simulink model "Transient_configuration_example_50_simscape"  (R2026a)
settings: Solver=ode23t  StopTime=120/60  EnableMultiTasking=on
undefined symbols (not defined in the file): Three_PhaseBreaker_class, Three_PhaseFault_class, Three_PhaseSeriesRLCLoad_class, Three_PhaseSource_class, Three_PhaseTransformer_1_class, Three_PhaseV_IMeasuremen_class
libraries: ee_lib x23, fl_lib x8, nesl_utility x8, eeRmsMeasurement x2
settings Model: Creator=Rodney Tan  LastModifiedBy=usuario
settings DebuggingCC: SaveWithParameterizedLinksMsg=none
settings SimscapeCC: SimscapeNormalizeSystem=off  SimscapeLogType=none  SimscapeLogDataHistory=5000.0

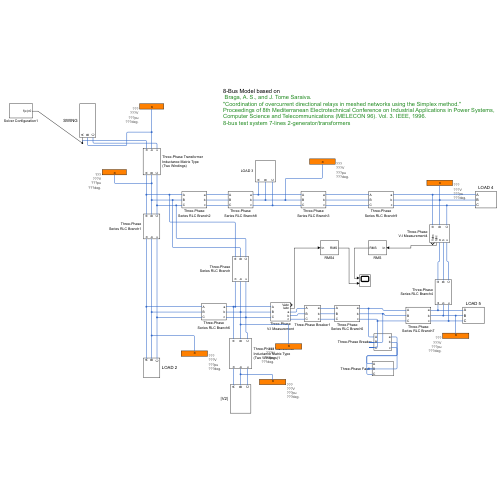
[thumbnail: Simulink's stored preview of the top-level diagram]
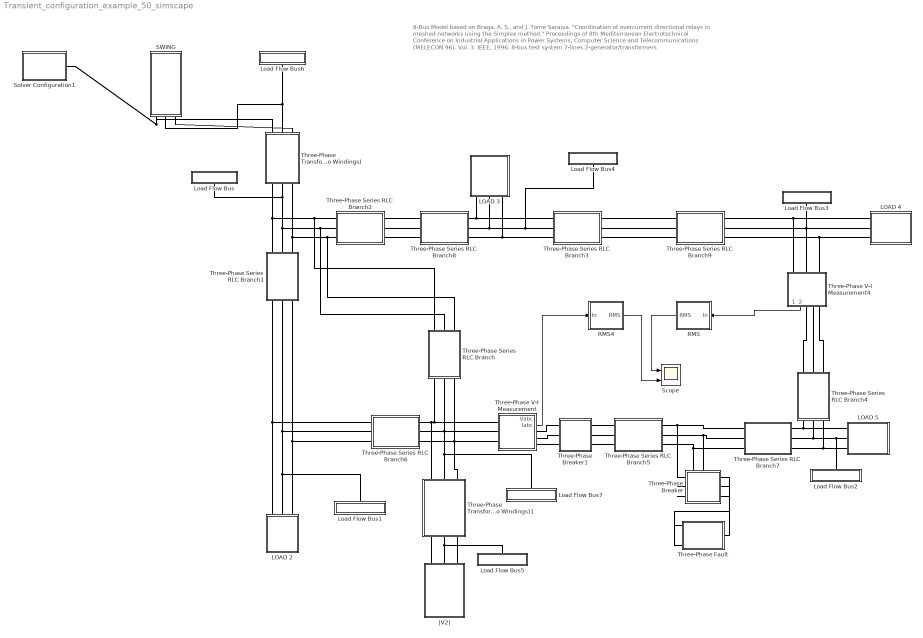
== system Transient_configuration_example_50_simscape ==
  note: 8-Bus Model based on
      | Braga, A. S., and J. Tome Saraiva.
      | "Coordination of overcurrent directional relays in meshed networks using the Simplex method."
      | Proceedings of 8th Mediterranean Electrotechnical Conference on Industrial Applications in Power Systems,
      | Computer Science and Telecommunications (MELECON 96). Vol. 3. IEEE, 1996.
      | 8-bus test system 7-lines 2-generator/transformers
  LOAD 2 : Subsystem
      settings: AttributesFormatString=\n  OpenFcn=elec.conv.unmask(gcb);
  LOAD 3 : Subsystem
      settings: AttributesFormatString=\n  OpenFcn=elec.conv.unmask(gcb);
  LOAD 4 : Subsystem
      settings: AttributesFormatString=\n  OpenFcn=elec.conv.unmask(gcb);
  LOAD 5 : Subsystem
      settings: AttributesFormatString=\n  OpenFcn=elec.conv.unmask(gcb);
  Load Flow Bus : Subsystem
      settings: OpenFcn=elec.conv.unmask(gcb);
      settings: AttributesFormatString=|
      | %<ID>
      | %<Vbase>V
      | %<VLF>pu
      | %<angleLF>deg.
  Load Flow Bus1 : Subsystem
      settings: OpenFcn=elec.conv.unmask(gcb);
      settings: AttributesFormatString=|
      | %<ID>
      | %<Vbase>V
      | %<VLF>pu
      | %<angleLF>deg.
  Load Flow Bus2 : Subsystem
      settings: OpenFcn=elec.conv.unmask(gcb);
      settings: AttributesFormatString=|
      | %<ID>
      | %<Vbase>V
      | %<VLF>pu
      | %<angleLF>deg.
  Load Flow Bus3 : Subsystem
      settings: OpenFcn=elec.conv.unmask(gcb);
      settings: AttributesFormatString=|
      | %<ID>
      | %<Vbase>V
      | %<VLF>pu
      | %<angleLF>deg.
  Load Flow Bus4 : Subsystem
      settings: OpenFcn=elec.conv.unmask(gcb);
      settings: AttributesFormatString=|
      | %<ID>
      | %<Vbase>V
      | %<VLF>pu
      | %<angleLF>deg.
  Load Flow Bus5 : Subsystem
      settings: OpenFcn=elec.conv.unmask(gcb);
      settings: AttributesFormatString=|
      | %<ID>
      | %<Vbase>V
      | %<VLF>pu
      | %<angleLF>deg.
  Load Flow Bus6 : Subsystem
      settings: OpenFcn=elec.conv.unmask(gcb);
      settings: AttributesFormatString=|
      | %<ID>
      | %<Vbase>V
      | %<VLF>pu
      | %<angleLF>deg.
  Load Flow Bus7 : Subsystem
      settings: OpenFcn=elec.conv.unmask(gcb);
      settings: AttributesFormatString=|
      | %<ID>
      | %<Vbase>V
      | %<VLF>pu
      | %<angleLF>deg.
  RMS : Subsystem
      settings: OpenFcn=elec.conv.unmask(gcb);
  RMS4 : Subsystem
      settings: OpenFcn=elec.conv.unmask(gcb);
  SWING : Subsystem
      settings: OpenFcn=elec.conv.unmask(gcb);
  Scope : Scope  NumInputPorts=2
      settings: ActiveDisplayYMinimum=-296.48253  ActiveDisplayYMaximum=2668.34273
  Solver Configuration1 : Subsystem  Priority=1  mask{TimeDomain=Continuous, UseLocalSolver=on, LocalSolverSampleTime=5e-05, LocalSolverChoice=NE_BACKWARD_EULER_ADVANCER, DoFixedCost=on, MaxNonlinIter=4}
      settings: OpenFcn=elec.conv.unmask(gcb);
      mask TypeOptions TimeDomain: Continuous | Discrete | Phasor
      mask TypeOptions UseLocalSolver:
      | Solver
      | Configuration/UseLocalSolver
      mask TypeOptions LocalSolverSampleTime:
      | Solver
      | Configuration/LocalSolverSampleTime
      mask TypeOptions LocalSolverChoice:
      | Solver
      | Configuration/LocalSolverChoice
      mask TypeOptions DoFixedCost:
      | Solver
      | Configuration/DoFixedCost
      mask TypeOptions MaxNonlinIter:
      | Solver
      | Configuration/MaxNonlinIter
  Three-Phase Series RLC Branch : Subsystem
      settings: AttributesFormatString=\n  OpenFcn=elec.conv.unmask(gcb);
  Three-Phase Series RLC Branch1 : Subsystem
      settings: AttributesFormatString=\n  OpenFcn=elec.conv.unmask(gcb);
  Three-Phase Series RLC Branch2 : Subsystem
      settings: AttributesFormatString=\n  OpenFcn=elec.conv.unmask(gcb);
  Three-Phase Series RLC Branch3 : Subsystem
      settings: AttributesFormatString=\n  OpenFcn=elec.conv.unmask(gcb);
  Three-Phase Series RLC Branch4 : Subsystem
      settings: AttributesFormatString=\n  OpenFcn=elec.conv.unmask(gcb);
  Three-Phase Series RLC Branch5 : Subsystem
      settings: AttributesFormatString=\n  OpenFcn=elec.conv.unmask(gcb);
  Three-Phase Series RLC Branch6 : Subsystem
      settings: AttributesFormatString=\n  OpenFcn=elec.conv.unmask(gcb);
  Three-Phase Series RLC Branch7 : Subsystem
      settings: AttributesFormatString=\n  OpenFcn=elec.conv.unmask(gcb);
  Three-Phase Series RLC Branch8 : Subsystem
      settings: AttributesFormatString=\n  OpenFcn=elec.conv.unmask(gcb);
  Three-Phase Series RLC Branch9 : Subsystem
      settings: AttributesFormatString=\n  OpenFcn=elec.conv.unmask(gcb);
  Three-Phase V-I Measurement : Subsystem
      settings: OpenFcn=elec.conv.unmask(gcb);
  Three-Phase V-I Measurement4 : Subsystem
      settings: OpenFcn=elec.conv.unmask(gcb);
  Three-Phase Breaker : Subsystem
      settings: OpenFcn=elec.conv.unmask(gcb);
  Three-Phase Breaker1 : Subsystem
      settings: OpenFcn=elec.conv.unmask(gcb);
  Three-Phase Fault : Subsystem
      settings: OpenFcn=elec.conv.unmask(gcb);
  Three-Phase Transformer Inductance Matrix Type (Two Windings) : Subsystem
      settings: OpenFcn=elec.conv.unmask(gcb);
  Three-Phase Transformer Inductance Matrix Type (Two Windings)1 : Subsystem
      settings: OpenFcn=elec.conv.unmask(gcb);
  |V2| : Subsystem
      settings: OpenFcn=elec.conv.unmask(gcb);
  wires:
  Three-Phase V-I Measurement4/2(Iabc) -> RMS/1(In)
  Three-Phase V-I Measurement/2(Iabc) -> RMS4/1(In)
  RMS4/1(RMS) -> Scope/2
  RMS/1(RMS) -> Scope/1
  connections:
  Three-Phase Transformer Inductance Matrix Type (Two Windings)/LConn2 -- Load Flow Bus/LConn1 -- Three-Phase Series RLC Branch/LConn2 -- Three-Phase Series RLC Branch2/LConn2 -- Three-Phase Series RLC Branch1/LConn2
  Three-Phase Transformer Inductance Matrix Type (Two Windings)/LConn1 -- Three-Phase Series RLC Branch/LConn1 -- Three-Phase Series RLC Branch2/LConn1 -- Three-Phase Series RLC Branch1/LConn1
  LOAD 2/LConn2 -- Load Flow Bus1/LConn1 -- Three-Phase Series RLC Branch6/LConn2 -- Three-Phase Series RLC Branch1/RConn2
  LOAD 2/LConn3 -- Three-Phase Series RLC Branch6/LConn3 -- Three-Phase Series RLC Branch1/RConn3
  Three-Phase Series RLC Branch1/LConn3 -- Three-Phase Series RLC Branch/LConn3 -- Three-Phase Series RLC Branch2/LConn3 -- Three-Phase Transformer Inductance Matrix Type (Two Windings)/LConn3
  Three-Phase Series RLC Branch3/LConn1 -- Three-Phase Series RLC Branch8/RConn1 -- LOAD 3/LConn1
  Three-Phase Series RLC Branch8/RConn2 -- LOAD 3/LConn2 -- Load Flow Bus4/LConn1 -- Three-Phase Series RLC Branch3/LConn2
  Three-Phase Series RLC Branch3/LConn3 -- Three-Phase Series RLC Branch8/RConn3 -- LOAD 3/LConn3
  LOAD 2/LConn1 -- Three-Phase Series RLC Branch6/LConn1 -- Three-Phase Series RLC Branch1/RConn1
  Load Flow Bus6/LConn1 -- SWING/RConn2 -- Three-Phase Transformer Inductance Matrix Type (Two Windings)/RConn2
  Three-Phase Transformer Inductance Matrix Type (Two Windings)1/RConn2 -- Load Flow Bus5/LConn1 -- |V2|/RConn2
  Three-Phase Transformer Inductance Matrix Type (Two Windings)1/RConn1 -- |V2|/RConn1
  |V2|/RConn3 -- Three-Phase Transformer Inductance Matrix Type (Two Windings)1/RConn3
  Three-Phase V-I Measurement/LConn2 -- Load Flow Bus7/LConn1 -- Three-Phase Transformer Inductance Matrix Type (Two Windings)1/LConn2 -- Three-Phase Series RLC Branch/RConn2 -- Three-Phase Series RLC Branch6/RConn2
  Three-Phase V-I Measurement/LConn1 -- Three-Phase Transformer Inductance Matrix Type (Two Windings)1/LConn1 -- Three-Phase Series RLC Branch6/RConn1 -- Three-Phase Series RLC Branch/RConn1
  Three-Phase V-I Measurement/LConn3 -- Three-Phase Transformer Inductance Matrix Type (Two Windings)1/LConn3 -- Three-Phase Series RLC Branch/RConn3 -- Three-Phase Series RLC Branch6/RConn3
  Three-Phase Series RLC Branch5/RConn2 -- Three-Phase Series RLC Branch7/LConn2 -- Three-Phase Breaker/LConn2
  Three-Phase Series RLC Branch5/RConn3 -- Three-Phase Breaker/LConn3 -- Three-Phase Series RLC Branch7/LConn3
  Three-Phase Series RLC Branch5/RConn1 -- Three-Phase Series RLC Branch7/LConn1 -- Three-Phase Breaker/LConn1
  LOAD 5/LConn2 -- Load Flow Bus2/LConn1 -- Three-Phase Series RLC Branch4/RConn2 -- Three-Phase Series RLC Branch7/RConn2
  LOAD 5/LConn1 -- Three-Phase Series RLC Branch4/RConn1 -- Three-Phase Series RLC Branch7/RConn1
  LOAD 5/LConn3 -- Three-Phase Series RLC Branch4/RConn3 -- Three-Phase Series RLC Branch7/RConn3
  Three-Phase Series RLC Branch4/LConn2 -- Three-Phase V-I Measurement4/RConn2
  Three-Phase Series RLC Branch4/LConn1 -- Three-Phase V-I Measurement4/RConn1
  Three-Phase Series RLC Branch4/LConn3 -- Three-Phase V-I Measurement4/RConn3
  LOAD 4/LConn2 -- Three-Phase Series RLC Branch9/RConn2 -- Load Flow Bus3/LConn1 -- Three-Phase V-I Measurement4/LConn2
  LOAD 4/LConn3 -- Three-Phase Series RLC Branch9/RConn3 -- Three-Phase V-I Measurement4/LConn3
  LOAD 4/LConn1 -- Three-Phase Series RLC Branch9/RConn1 -- Three-Phase V-I Measurement4/LConn1
  Three-Phase Series RLC Branch2/RConn2 -- Three-Phase Series RLC Branch8/LConn2
  Three-Phase Series RLC Branch2/RConn3 -- Three-Phase Series RLC Branch8/LConn3
  Three-Phase Series RLC Branch2/RConn1 -- Three-Phase Series RLC Branch8/LConn1
  Three-Phase Series RLC Branch3/RConn3 -- Three-Phase Series RLC Branch9/LConn3
  Three-Phase Series RLC Branch3/RConn2 -- Three-Phase Series RLC Branch9/LConn2
  Three-Phase Series RLC Branch3/RConn1 -- Three-Phase Series RLC Branch9/LConn1
  Three-Phase Breaker/RConn3 -- Three-Phase Fault/LConn3
  Three-Phase Breaker/RConn2 -- Three-Phase Fault/LConn2
  Three-Phase Breaker/RConn1 -- Three-Phase Fault/LConn1
  Three-Phase Breaker1/RConn1 -- Three-Phase Series RLC Branch5/LConn1
  Three-Phase Breaker1/RConn2 -- Three-Phase Series RLC Branch5/LConn2
  Three-Phase Breaker1/RConn3 -- Three-Phase Series RLC Branch5/LConn3
  Three-Phase V-I Measurement/RConn1 -- Three-Phase Breaker1/LConn1
  Three-Phase V-I Measurement/RConn2 -- Three-Phase Breaker1/LConn2
  Three-Phase V-I Measurement/RConn3 -- Three-Phase Breaker1/LConn3
  SWING/RConn3 -- Three-Phase Transformer Inductance Matrix Type (Two Windings)/RConn3
  Three-Phase Transformer Inductance Matrix Type (Two Windings)/RConn1 -- SWING/RConn1 -- Solver Configuration1/RConn1

== system Transient_configuration_example_50_simscape/LOAD 2 ==
  Electrical Reference : fl_lib/Electrical/Electrical Elements/Electrical Reference
  Wye-Connected Load : ee_lib/Passive/RLC Assemblies/Wye-Connected Load  port_option=ee.enum.threePhasePort.expanded  parameterization=2  component_structure=4  component_structure_PQ=4  R=1 Ohm  L=0.001 H  C=1e-6 F  VRated=151341 V  FRated=60 Hz  P=40000000 W  Qpos=20000000 V*A  Qneg=Three_PhaseSeriesRLCLoad_class(0).objParamMappingDerived.NewDerivedParam.Qneg V*A  R_parasitic=1e-6 Ohm  G_parasitic=1e-6 1/Ohm  R_parasitic_PQ=1e-6 Ohm  G_parasitic_PQ=1e-6 1/Ohm  Vmag0=151341 V  Vang0=0 deg  Freq0=60 Hz  IL_specify=on  IL_priority=High  IL=[ 0 0 0 ] A  IL_nominal_specify=off  IL_nominal_value=1  IL_nominal_unit=A  VC_specify=on  VC_priority=High  VC=[ 0 0 0 ] V  VC_nominal_specify=off  VC_nominal_value=1  VC_nominal_unit=V
  A : PMIOPort  Side=Left
  B : PMIOPort  Port=2  Side=Left
  C : PMIOPort  Port=3  Side=Left
  connections:
  Electrical Reference/LConn1 -- Wye-Connected Load/RConn1
  Wye-Connected Load/LConn3 -- C/RConn1
  Wye-Connected Load/LConn1 -- A/RConn1
  Wye-Connected Load/LConn2 -- B/RConn1

== system Transient_configuration_example_50_simscape/LOAD 3 ==
  Electrical Reference : fl_lib/Electrical/Electrical Elements/Electrical Reference
  Wye-Connected Load : ee_lib/Passive/RLC Assemblies/Wye-Connected Load  port_option=ee.enum.threePhasePort.expanded  parameterization=2  component_structure=4  component_structure_PQ=4  R=1 Ohm  L=0.001 H  C=1e-6 F  VRated=148678.8 V  FRated=60 Hz  P=60000000 W  Qpos=40000000 V*A  Qneg=Three_PhaseSeriesRLCLoad_class(0).objParamMappingDerived.NewDerivedParam.Qneg V*A  R_parasitic=1e-6 Ohm  G_parasitic=1e-6 1/Ohm  R_parasitic_PQ=1e-6 Ohm  G_parasitic_PQ=1e-6 1/Ohm  Vmag0=148678.8 V  Vang0=0 deg  Freq0=60 Hz  IL_specify=on  IL_priority=High  IL=[ 0 0 0 ] A  IL_nominal_specify=off  IL_nominal_value=1  IL_nominal_unit=A  VC_specify=on  VC_priority=High  VC=[ 0 0 0 ] V  VC_nominal_specify=off  VC_nominal_value=1  VC_nominal_unit=V
  A : PMIOPort  Side=Left
  B : PMIOPort  Port=2  Side=Left
  C : PMIOPort  Port=3  Side=Left
  connections:
  Electrical Reference/LConn1 -- Wye-Connected Load/RConn1
  Wye-Connected Load/LConn3 -- C/RConn1
  Wye-Connected Load/LConn1 -- A/RConn1
  Wye-Connected Load/LConn2 -- B/RConn1

== system Transient_configuration_example_50_simscape/LOAD 4 ==
  Electrical Reference : fl_lib/Electrical/Electrical Elements/Electrical Reference
  Wye-Connected Load : ee_lib/Passive/RLC Assemblies/Wye-Connected Load  port_option=ee.enum.threePhasePort.expanded  parameterization=2  component_structure=4  component_structure_PQ=4  R=1 Ohm  L=0.001 H  C=1e-6 F  VRated=148827 V  FRated=60 Hz  P=70000000 W  Qpos=40000000 V*A  Qneg=Three_PhaseSeriesRLCLoad_class(0).objParamMappingDerived.NewDerivedParam.Qneg V*A  R_parasitic=1e-6 Ohm  G_parasitic=1e-6 1/Ohm  R_parasitic_PQ=1e-6 Ohm  G_parasitic_PQ=1e-6 1/Ohm  Vmag0=148827 V  Vang0=0 deg  Freq0=60 Hz  IL_specify=on  IL_priority=High  IL=[ 0 0 0 ] A  IL_nominal_specify=off  IL_nominal_value=1  IL_nominal_unit=A  VC_specify=on  VC_priority=High  VC=[ 0 0 0 ] V  VC_nominal_specify=off  VC_nominal_value=1  VC_nominal_unit=V
  A : PMIOPort  Side=Left
  B : PMIOPort  Port=2  Side=Left
  C : PMIOPort  Port=3  Side=Left
  connections:
  Electrical Reference/LConn1 -- Wye-Connected Load/RConn1
  Wye-Connected Load/LConn3 -- C/RConn1
  Wye-Connected Load/LConn1 -- A/RConn1
  Wye-Connected Load/LConn2 -- B/RConn1

== system Transient_configuration_example_50_simscape/LOAD 5 ==
  Electrical Reference : fl_lib/Electrical/Electrical Elements/Electrical Reference
  Wye-Connected Load : ee_lib/Passive/RLC Assemblies/Wye-Connected Load  port_option=ee.enum.threePhasePort.expanded  parameterization=2  component_structure=4  component_structure_PQ=4  R=1 Ohm  L=0.001 H  C=1e-6 F  VRated=150411 V  FRated=60 Hz  P=70000000 W  Qpos=50000000 V*A  Qneg=Three_PhaseSeriesRLCLoad_class(0).objParamMappingDerived.NewDerivedParam.Qneg V*A  R_parasitic=1e-6 Ohm  G_parasitic=1e-6 1/Ohm  R_parasitic_PQ=1e-6 Ohm  G_parasitic_PQ=1e-6 1/Ohm  Vmag0=150411 V  Vang0=0 deg  Freq0=60 Hz  IL_specify=on  IL_priority=High  IL=[ 0 0 0 ] A  IL_nominal_specify=off  IL_nominal_value=1  IL_nominal_unit=A  VC_specify=on  VC_priority=High  VC=[ 0 0 0 ] V  VC_nominal_specify=off  VC_nominal_value=1  VC_nominal_unit=V
  A : PMIOPort  Side=Left
  B : PMIOPort  Port=2  Side=Left
  C : PMIOPort  Port=3  Side=Left
  connections:
  Electrical Reference/LConn1 -- Wye-Connected Load/RConn1
  Wye-Connected Load/LConn3 -- C/RConn1
  Wye-Connected Load/LConn1 -- A/RConn1
  Wye-Connected Load/LConn2 -- B/RConn1

== system Transient_configuration_example_50_simscape/Load Flow Bus ==
  a : PMIOPort  Side=Left

== system Transient_configuration_example_50_simscape/Load Flow Bus1 ==
  a : PMIOPort  Side=Left

== system Transient_configuration_example_50_simscape/Load Flow Bus2 ==
  a : PMIOPort  Side=Left

== system Transient_configuration_example_50_simscape/Load Flow Bus3 ==
  a : PMIOPort  Side=Left

== system Transient_configuration_example_50_simscape/Load Flow Bus4 ==
  a : PMIOPort  Side=Left

== system Transient_configuration_example_50_simscape/Load Flow Bus5 ==
  a : PMIOPort  Side=Left

== system Transient_configuration_example_50_simscape/Load Flow Bus6 ==
  a : PMIOPort  Side=Left

== system Transient_configuration_example_50_simscape/Load Flow Bus7 ==
  a : PMIOPort  Side=Left

== system Transient_configuration_example_50_simscape/RMS ==
  In : Inport
  RMS Measurement : eeRmsMeasurement/RMS Measurement  LabelModeActiveChoice=Total  F=60  SpecifyHarmonics=off  K=1  Ts=0
  RMS : Outport  VectorParamsAs1DForOutWhenUnconnected=off
  wires:
  RMS Measurement/1 -> RMS/1
  In/1 -> RMS Measurement/1

== system Transient_configuration_example_50_simscape/RMS4 ==
  In : Inport
  RMS Measurement : eeRmsMeasurement/RMS Measurement  LabelModeActiveChoice=Total  F=60  SpecifyHarmonics=off  K=1  Ts=0
  RMS : Outport  VectorParamsAs1DForOutWhenUnconnected=off
  wires:
  RMS Measurement/1 -> RMS/1
  In/1 -> RMS Measurement/1

== system Transient_configuration_example_50_simscape/SWING ==
  Electrical Reference : fl_lib/Electrical/Electrical Elements/Electrical Reference
  Voltage Source : ee_lib/Sources/Voltage Source (Three-Phase)  vline_rms=10288.4 V  shift=-8.3669 deg  freq=60 Hz  impedance_option=3  SShortCircuit=100000000 V*A  XR=7  R=Three_PhaseSource_class(10288.4,60,0,0.00026525198938992,100000000,10000,7,'on','off').objParamMappingDerived.NewDerivedParam.R Ohm  L=Three_PhaseSource_class(10288.4,60,0,0.00026525198938992,100000000,10000,7,'on','off').objParamMappingDerived.NewDerivedParam.L H  harmonic_option=0  harmonic_orders=[5, 7, 11, 13]  harmonic_ratios=[.1, .1, .1, .1]  G_parasitic=0 1/Ohm  I_specify=off  I_priority=None  I=[ 0 0 0 ] A  I_nominal_specify=off  I_nominal_value=1  I_nominal_unit=A
  A : PMIOPort  Side=Right
  B : PMIOPort  Port=2  Side=Right
  C : PMIOPort  Port=3  Side=Right
  connections:
  Voltage Source/RConn2 -- B/RConn1
  Voltage Source/RConn1 -- A/RConn1
  Voltage Source/RConn3 -- C/RConn1
  Electrical Reference/LConn1 -- Voltage Source/LConn1

== system Transient_configuration_example_50_simscape/Solver Configuration1 ==
  Solver Configuration : nesl_utility/Solver Configuration  PhysicalDomain=network_engine_domain  SubClassName=solver  LeftPortType=input  RightPortType=generic  Tones=[]  Harmonics=[]  SimulateNoise=off  Profile=off  UseLocalSampling=off  EnableSwitchedLinearOptims=on  FrequencyDomain=off  UseCCode=off  RelTol=0.001  AbsTol=1e-06  MinStep=1e-09  ToWorkspace=off  RevertToSquareIcSolve=off  NumHomotopyIterations=100  PhasorMode=off  PhasorModeNumHarmonics=1  ConsistencySolver=NEWTON_FTOL  CanonicalOrdering=UNORDERED  OptimizeIntermediates=UNOPTIMIZED  IndexReductionMethod=DerivativeReplacement  DoDC=off  ResidualTolerance=1e-09  ConsistencyTolSource=GLOBAL  ConsistencyAbsTol=0.001  ConsistencyRelTol=0.001  ConsistencyTolFactor=0.001  UseLocalSolver=on  LocalSolverChoice=NE_BACKWARD_EULER_ADVANCER  ResolveIndetEquations=off  FunctionEvalNumThread=1  LocalSolverSampleTime=LocalSolverSampleTime  DoFixedCost=on  MaxNonlinIter=MaxNonlinIter  MaxModeIter=2  ComputeImpulses=off  ImpulseIterations=1  LinearAlgebra=auto  LinearAlgebraNumThread=0  EquationFormulation=NE_TIME_EF  DelaysMemoryBudget=1024  AutomaticFiltering=on  FilteringTimeConstant=0.001  PartitionStorageMethod=AS_NEEDED  PartitionMemoryBudget=1024  PartitionMethod=FAST  MultibodyUseLocalSolver=off  MultibodyLocalSolverChoice=ODE1  MultibodyLocalSolverSampleTime=0.001
  f(x)=0 : PMIOPort  Side=Right
  connections:
  f(x)=0/RConn1 -- Solver Configuration/RConn1

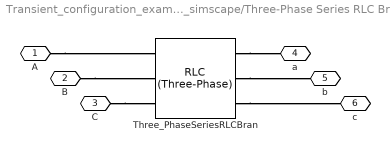
== system Transient_configuration_example_50_simscape/Three-Phase Series RLC Branch ==
  Three_PhaseSeriesRLCBran : ee_lib/Passive/RLC Assemblies/RLC (Three-Phase)  port_option=ee.enum.threePhasePort.expanded  component_structure=4  R=0.5 Ohm  L=0.013263 H  C=1e-06 F  R_parasitic=1e-6 Ohm  G_parasitic=1e-6 1/Ohm  IL_specify=on  IL_priority=High  IL=[0, 0, 0] A  IL_nominal_specify=off  IL_nominal_value=1  IL_nominal_unit=A  VC_specify=on  VC_priority=High  VC=[0, 0, 0] V  VC_nominal_specify=off  VC_nominal_value=1  VC_nominal_unit=V
  A : PMIOPort  Side=Left
  B : PMIOPort  Port=2  Side=Left
  C : PMIOPort  Port=3  Side=Left
  a : PMIOPort  Port=4  Side=Right
  b : PMIOPort  Port=5  Side=Right
  c : PMIOPort  Port=6  Side=Right
  connections:
  Three_PhaseSeriesRLCBran/RConn3 -- c/RConn1
  Three_PhaseSeriesRLCBran/RConn2 -- b/RConn1
  Three_PhaseSeriesRLCBran/RConn1 -- a/RConn1
  C/RConn1 -- Three_PhaseSeriesRLCBran/LConn3
  B/RConn1 -- Three_PhaseSeriesRLCBran/LConn2
  A/RConn1 -- Three_PhaseSeriesRLCBran/LConn1

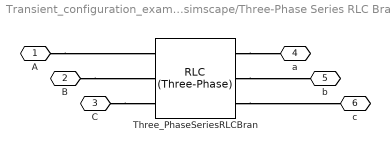
== system Transient_configuration_example_50_simscape/Three-Phase Series RLC Branch1 ==
  Three_PhaseSeriesRLCBran : ee_lib/Passive/RLC Assemblies/RLC (Three-Phase)  port_option=ee.enum.threePhasePort.expanded  component_structure=4  R=0.4 Ohm  L=0.013263 H  C=1e-06 F  R_parasitic=1e-6 Ohm  G_parasitic=1e-6 1/Ohm  IL_specify=on  IL_priority=High  IL=[0, 0, 0] A  IL_nominal_specify=off  IL_nominal_value=1  IL_nominal_unit=A  VC_specify=on  VC_priority=High  VC=[0, 0, 0] V  VC_nominal_specify=off  VC_nominal_value=1  VC_nominal_unit=V
  A : PMIOPort  Side=Left
  B : PMIOPort  Port=2  Side=Left
  C : PMIOPort  Port=3  Side=Left
  a : PMIOPort  Port=4  Side=Right
  b : PMIOPort  Port=5  Side=Right
  c : PMIOPort  Port=6  Side=Right
  connections:
  Three_PhaseSeriesRLCBran/RConn3 -- c/RConn1
  Three_PhaseSeriesRLCBran/RConn2 -- b/RConn1
  Three_PhaseSeriesRLCBran/RConn1 -- a/RConn1
  C/RConn1 -- Three_PhaseSeriesRLCBran/LConn3
  B/RConn1 -- Three_PhaseSeriesRLCBran/LConn2
  A/RConn1 -- Three_PhaseSeriesRLCBran/LConn1

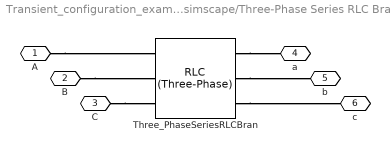
== system Transient_configuration_example_50_simscape/Three-Phase Series RLC Branch2 ==
  Three_PhaseSeriesRLCBran : ee_lib/Passive/RLC Assemblies/RLC (Three-Phase)  port_option=ee.enum.threePhasePort.expanded  component_structure=4  R=0.1995 Ohm  L=0.0066286 H  C=1e-06 F  R_parasitic=1e-6 Ohm  G_parasitic=1e-6 1/Ohm  IL_specify=on  IL_priority=High  IL=[0, 0, 0] A  IL_nominal_specify=off  IL_nominal_value=1  IL_nominal_unit=A  VC_specify=on  VC_priority=High  VC=[0, 0, 0] V  VC_nominal_specify=off  VC_nominal_value=1  VC_nominal_unit=V
  A : PMIOPort  Side=Left
  B : PMIOPort  Port=2  Side=Left
  C : PMIOPort  Port=3  Side=Left
  a : PMIOPort  Port=4  Side=Right
  b : PMIOPort  Port=5  Side=Right
  c : PMIOPort  Port=6  Side=Right
  connections:
  Three_PhaseSeriesRLCBran/RConn3 -- c/RConn1
  Three_PhaseSeriesRLCBran/RConn2 -- b/RConn1
  Three_PhaseSeriesRLCBran/RConn1 -- a/RConn1
  C/RConn1 -- Three_PhaseSeriesRLCBran/LConn3
  B/RConn1 -- Three_PhaseSeriesRLCBran/LConn2
  A/RConn1 -- Three_PhaseSeriesRLCBran/LConn1

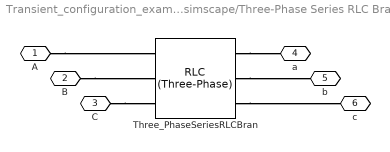
== system Transient_configuration_example_50_simscape/Three-Phase Series RLC Branch3 ==
  Three_PhaseSeriesRLCBran : ee_lib/Passive/RLC Assemblies/RLC (Three-Phase)  port_option=ee.enum.threePhasePort.expanded  component_structure=4  R=0.2 Ohm  L=0.0059735 H  C=1e-06 F  R_parasitic=1e-6 Ohm  G_parasitic=1e-6 1/Ohm  IL_specify=on  IL_priority=High  IL=[0, 0, 0] A  IL_nominal_specify=off  IL_nominal_value=1  IL_nominal_unit=A  VC_specify=on  VC_priority=High  VC=[0, 0, 0] V  VC_nominal_specify=off  VC_nominal_value=1  VC_nominal_unit=V
  A : PMIOPort  Side=Left
  B : PMIOPort  Port=2  Side=Left
  C : PMIOPort  Port=3  Side=Left
  a : PMIOPort  Port=4  Side=Right
  b : PMIOPort  Port=5  Side=Right
  c : PMIOPort  Port=6  Side=Right
  connections:
  Three_PhaseSeriesRLCBran/RConn3 -- c/RConn1
  Three_PhaseSeriesRLCBran/RConn2 -- b/RConn1
  Three_PhaseSeriesRLCBran/RConn1 -- a/RConn1
  C/RConn1 -- Three_PhaseSeriesRLCBran/LConn3
  B/RConn1 -- Three_PhaseSeriesRLCBran/LConn2
  A/RConn1 -- Three_PhaseSeriesRLCBran/LConn1

== system Transient_configuration_example_50_simscape/Three-Phase Series RLC Branch4 ==
  Three_PhaseSeriesRLCBran : ee_lib/Passive/RLC Assemblies/RLC (Three-Phase)  port_option=ee.enum.threePhasePort.expanded  component_structure=4  R=0.5 Ohm  L=0.011936 H  C=1e-06 F  R_parasitic=1e-6 Ohm  G_parasitic=1e-6 1/Ohm  IL_specify=on  IL_priority=High  IL=[0, 0, 0] A  IL_nominal_specify=off  IL_nominal_value=1  IL_nominal_unit=A  VC_specify=on  VC_priority=High  VC=[0, 0, 0] V  VC_nominal_specify=off  VC_nominal_value=1  VC_nominal_unit=V
  A : PMIOPort  Side=Left
  B : PMIOPort  Port=2  Side=Left
  C : PMIOPort  Port=3  Side=Left
  a : PMIOPort  Port=4  Side=Right
  b : PMIOPort  Port=5  Side=Right
  c : PMIOPort  Port=6  Side=Right
  connections:
  Three_PhaseSeriesRLCBran/RConn3 -- c/RConn1
  Three_PhaseSeriesRLCBran/RConn2 -- b/RConn1
  Three_PhaseSeriesRLCBran/RConn1 -- a/RConn1
  C/RConn1 -- Three_PhaseSeriesRLCBran/LConn3
  B/RConn1 -- Three_PhaseSeriesRLCBran/LConn2
  A/RConn1 -- Three_PhaseSeriesRLCBran/LConn1

== system Transient_configuration_example_50_simscape/Three-Phase Series RLC Branch5 ==
  Three_PhaseSeriesRLCBran : ee_lib/Passive/RLC Assemblies/RLC (Three-Phase)  port_option=ee.enum.threePhasePort.expanded  component_structure=4  R=0.039154 Ohm  L=0.00094395 H  C=1e-06 F  R_parasitic=1e-6 Ohm  G_parasitic=1e-6 1/Ohm  IL_specify=on  IL_priority=High  IL=[0, 0, 0] A  IL_nominal_specify=off  IL_nominal_value=1  IL_nominal_unit=A  VC_specify=on  VC_priority=High  VC=[0, 0, 0] V  VC_nominal_specify=off  VC_nominal_value=1  VC_nominal_unit=V
  A : PMIOPort  Side=Left
  B : PMIOPort  Port=2  Side=Left
  C : PMIOPort  Port=3  Side=Left
  a : PMIOPort  Port=4  Side=Right
  b : PMIOPort  Port=5  Side=Right
  c : PMIOPort  Port=6  Side=Right
  connections:
  Three_PhaseSeriesRLCBran/RConn3 -- c/RConn1
  Three_PhaseSeriesRLCBran/RConn2 -- b/RConn1
  Three_PhaseSeriesRLCBran/RConn1 -- a/RConn1
  C/RConn1 -- Three_PhaseSeriesRLCBran/LConn3
  B/RConn1 -- Three_PhaseSeriesRLCBran/LConn2
  A/RConn1 -- Three_PhaseSeriesRLCBran/LConn1

== system Transient_configuration_example_50_simscape/Three-Phase Series RLC Branch6 ==
  Three_PhaseSeriesRLCBran : ee_lib/Passive/RLC Assemblies/RLC (Three-Phase)  port_option=ee.enum.threePhasePort.expanded  component_structure=4  R=0.396 Ohm  L=0.011936 H  C=1e-06 F  R_parasitic=1e-6 Ohm  G_parasitic=1e-6 1/Ohm  IL_specify=on  IL_priority=High  IL=[0, 0, 0] A  IL_nominal_specify=off  IL_nominal_value=1  IL_nominal_unit=A  VC_specify=on  VC_priority=High  VC=[0, 0, 0] V  VC_nominal_specify=off  VC_nominal_value=1  VC_nominal_unit=V
  A : PMIOPort  Side=Left
  B : PMIOPort  Port=2  Side=Left
  C : PMIOPort  Port=3  Side=Left
  a : PMIOPort  Port=4  Side=Right
  b : PMIOPort  Port=5  Side=Right
  c : PMIOPort  Port=6  Side=Right
  connections:
  Three_PhaseSeriesRLCBran/RConn3 -- c/RConn1
  Three_PhaseSeriesRLCBran/RConn2 -- b/RConn1
  Three_PhaseSeriesRLCBran/RConn1 -- a/RConn1
  C/RConn1 -- Three_PhaseSeriesRLCBran/LConn3
  B/RConn1 -- Three_PhaseSeriesRLCBran/LConn2
  A/RConn1 -- Three_PhaseSeriesRLCBran/LConn1

== system Transient_configuration_example_50_simscape/Three-Phase Series RLC Branch7 ==
  Three_PhaseSeriesRLCBran : ee_lib/Passive/RLC Assemblies/RLC (Three-Phase)  port_option=ee.enum.threePhasePort.expanded  component_structure=4  R=0.45585 Ohm  L=0.01099 H  C=1e-06 F  R_parasitic=1e-6 Ohm  G_parasitic=1e-6 1/Ohm  IL_specify=on  IL_priority=High  IL=[0, 0, 0] A  IL_nominal_specify=off  IL_nominal_value=1  IL_nominal_unit=A  VC_specify=on  VC_priority=High  VC=[0, 0, 0] V  VC_nominal_specify=off  VC_nominal_value=1  VC_nominal_unit=V
  A : PMIOPort  Side=Left
  B : PMIOPort  Port=2  Side=Left
  C : PMIOPort  Port=3  Side=Left
  a : PMIOPort  Port=4  Side=Right
  b : PMIOPort  Port=5  Side=Right
  c : PMIOPort  Port=6  Side=Right
  connections:
  Three_PhaseSeriesRLCBran/RConn3 -- c/RConn1
  Three_PhaseSeriesRLCBran/RConn2 -- b/RConn1
  Three_PhaseSeriesRLCBran/RConn1 -- a/RConn1
  C/RConn1 -- Three_PhaseSeriesRLCBran/LConn3
  B/RConn1 -- Three_PhaseSeriesRLCBran/LConn2
  A/RConn1 -- Three_PhaseSeriesRLCBran/LConn1

== system Transient_configuration_example_50_simscape/Three-Phase Series RLC Branch8 ==
  Three_PhaseSeriesRLCBran : ee_lib/Passive/RLC Assemblies/RLC (Three-Phase)  port_option=ee.enum.threePhasePort.expanded  component_structure=4  R=0.1995 Ohm  L=0.0066286 H  C=1e-06 F  R_parasitic=1e-6 Ohm  G_parasitic=1e-6 1/Ohm  IL_specify=on  IL_priority=High  IL=[0, 0, 0] A  IL_nominal_specify=off  IL_nominal_value=1  IL_nominal_unit=A  VC_specify=on  VC_priority=High  VC=[0, 0, 0] V  VC_nominal_specify=off  VC_nominal_value=1  VC_nominal_unit=V
  A : PMIOPort  Side=Left
  B : PMIOPort  Port=2  Side=Left
  C : PMIOPort  Port=3  Side=Left
  a : PMIOPort  Port=4  Side=Right
  b : PMIOPort  Port=5  Side=Right
  c : PMIOPort  Port=6  Side=Right
  connections:
  Three_PhaseSeriesRLCBran/RConn3 -- c/RConn1
  Three_PhaseSeriesRLCBran/RConn2 -- b/RConn1
  Three_PhaseSeriesRLCBran/RConn1 -- a/RConn1
  C/RConn1 -- Three_PhaseSeriesRLCBran/LConn3
  B/RConn1 -- Three_PhaseSeriesRLCBran/LConn2
  A/RConn1 -- Three_PhaseSeriesRLCBran/LConn1

== system Transient_configuration_example_50_simscape/Three-Phase Series RLC Branch9 ==
  Three_PhaseSeriesRLCBran : ee_lib/Passive/RLC Assemblies/RLC (Three-Phase)  port_option=ee.enum.threePhasePort.expanded  component_structure=4  R=0.2 Ohm  L=0.0059735 H  C=1e-06 F  R_parasitic=1e-6 Ohm  G_parasitic=1e-6 1/Ohm  IL_specify=on  IL_priority=High  IL=[0, 0, 0] A  IL_nominal_specify=off  IL_nominal_value=1  IL_nominal_unit=A  VC_specify=on  VC_priority=High  VC=[0, 0, 0] V  VC_nominal_specify=off  VC_nominal_value=1  VC_nominal_unit=V
  A : PMIOPort  Side=Left
  B : PMIOPort  Port=2  Side=Left
  C : PMIOPort  Port=3  Side=Left
  a : PMIOPort  Port=4  Side=Right
  b : PMIOPort  Port=5  Side=Right
  c : PMIOPort  Port=6  Side=Right
  connections:
  Three_PhaseSeriesRLCBran/RConn3 -- c/RConn1
  Three_PhaseSeriesRLCBran/RConn2 -- b/RConn1
  Three_PhaseSeriesRLCBran/RConn1 -- a/RConn1
  C/RConn1 -- Three_PhaseSeriesRLCBran/LConn3
  B/RConn1 -- Three_PhaseSeriesRLCBran/LConn2
  A/RConn1 -- Three_PhaseSeriesRLCBran/LConn1

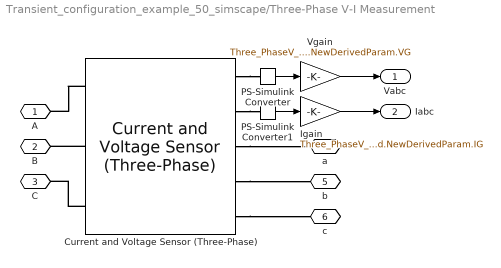
== system Transient_configuration_example_50_simscape/Three-Phase V-I Measurement ==
  Current and Voltage Sensor (Three-Phase) : ee_lib/Sensors & Transducers/Current and Voltage Sensor (Three-Phase)  port_option=ee.enum.threePhasePort.expanded  vMeasurementType=2  outputUnit=2  SRated=100000000 V*A  VRated=500000 V  I_specify=off  I_priority=None  I=[ 0 0 0 ] A  I_nominal_specify=off  I_nominal_value=1  I_nominal_unit=A  V_specify=off  V_priority=None  V=[ 0 0 0 ] V  V_nominal_specify=off  V_nominal_value=1  V_nominal_unit=V
  Igain : Gain  Gain=Three_PhaseV_IMeasuremen_class('phase-to-ground','yes','off','off','off',100000000,500000).objParamMappingDerived.NewDerivedParam.IG
  PS-Simulink Converter : nesl_utility/PS-Simulink Converter  PhysicalDomain=network_engine_domain  SubClassName=ps_output  LeftPortType=input  RightPortType=output  PseudoPeriodic=off  Frequencies=[]  VectorFormat=1-D array  Unit=1  AffineConversion=off
  PS-Simulink Converter1 : nesl_utility/PS-Simulink Converter  PhysicalDomain=network_engine_domain  SubClassName=ps_output  LeftPortType=input  RightPortType=output  PseudoPeriodic=off  Frequencies=[]  VectorFormat=1-D array  Unit=1  AffineConversion=off
  Vgain : Gain  Gain=Three_PhaseV_IMeasuremen_class('phase-to-ground','yes','off','off','off',100000000,500000).objParamMappingDerived.NewDerivedParam.VG
  A : PMIOPort  Side=Left
  B : PMIOPort  Port=2  Side=Left
  C : PMIOPort  Port=3  Side=Left
  a : PMIOPort  Port=4  Side=Right
  b : PMIOPort  Port=5  Side=Right
  c : PMIOPort  Port=6  Side=Right
  Vabc : Outport  VectorParamsAs1DForOutWhenUnconnected=off
  Iabc : Outport  Port=2  VectorParamsAs1DForOutWhenUnconnected=off
  wires:
  Igain/1 -> Iabc/1
  Vgain/1 -> Vabc/1
  PS-Simulink Converter1/1 -> Igain/1
  PS-Simulink Converter/1 -> Vgain/1
  connections:
  Current and Voltage Sensor (Three-Phase)/RConn1 -- PS-Simulink Converter/LConn1
  Current and Voltage Sensor (Three-Phase)/RConn2 -- PS-Simulink Converter1/LConn1
  Current and Voltage Sensor (Three-Phase)/RConn5 -- c/RConn1
  Current and Voltage Sensor (Three-Phase)/RConn4 -- b/RConn1
  Current and Voltage Sensor (Three-Phase)/RConn3 -- a/RConn1
  Current and Voltage Sensor (Three-Phase)/LConn3 -- C/RConn1
  Current and Voltage Sensor (Three-Phase)/LConn1 -- A/RConn1
  Current and Voltage Sensor (Three-Phase)/LConn2 -- B/RConn1

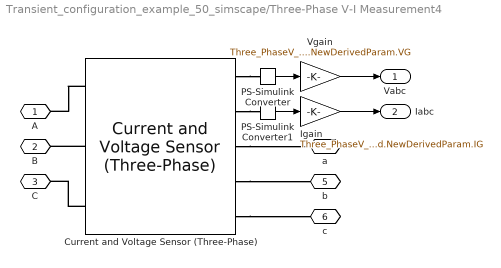
== system Transient_configuration_example_50_simscape/Three-Phase V-I Measurement4 ==
  Current and Voltage Sensor (Three-Phase) : ee_lib/Sensors & Transducers/Current and Voltage Sensor (Three-Phase)  port_option=ee.enum.threePhasePort.expanded  vMeasurementType=2  outputUnit=2  SRated=100000000 V*A  VRated=500000 V  I_specify=off  I_priority=None  I=[ 0 0 0 ] A  I_nominal_specify=off  I_nominal_value=1  I_nominal_unit=A  V_specify=off  V_priority=None  V=[ 0 0 0 ] V  V_nominal_specify=off  V_nominal_value=1  V_nominal_unit=V
  Igain : Gain  Gain=Three_PhaseV_IMeasuremen_class('phase-to-ground','yes','off','off','off',100000000,500000).objParamMappingDerived.NewDerivedParam.IG
  PS-Simulink Converter : nesl_utility/PS-Simulink Converter  PhysicalDomain=network_engine_domain  SubClassName=ps_output  LeftPortType=input  RightPortType=output  PseudoPeriodic=off  Frequencies=[]  VectorFormat=1-D array  Unit=1  AffineConversion=off
  PS-Simulink Converter1 : nesl_utility/PS-Simulink Converter  PhysicalDomain=network_engine_domain  SubClassName=ps_output  LeftPortType=input  RightPortType=output  PseudoPeriodic=off  Frequencies=[]  VectorFormat=1-D array  Unit=1  AffineConversion=off
  Vgain : Gain  Gain=Three_PhaseV_IMeasuremen_class('phase-to-ground','yes','off','off','off',100000000,500000).objParamMappingDerived.NewDerivedParam.VG
  A : PMIOPort  Side=Left
  B : PMIOPort  Port=2  Side=Left
  C : PMIOPort  Port=3  Side=Left
  a : PMIOPort  Port=4  Side=Right
  b : PMIOPort  Port=5  Side=Right
  c : PMIOPort  Port=6  Side=Right
  Vabc : Outport  VectorParamsAs1DForOutWhenUnconnected=off
  Iabc : Outport  Port=2  VectorParamsAs1DForOutWhenUnconnected=off
  wires:
  Igain/1 -> Iabc/1
  Vgain/1 -> Vabc/1
  PS-Simulink Converter1/1 -> Igain/1
  PS-Simulink Converter/1 -> Vgain/1
  connections:
  Current and Voltage Sensor (Three-Phase)/RConn1 -- PS-Simulink Converter/LConn1
  Current and Voltage Sensor (Three-Phase)/RConn2 -- PS-Simulink Converter1/LConn1
  Current and Voltage Sensor (Three-Phase)/RConn5 -- c/RConn1
  Current and Voltage Sensor (Three-Phase)/RConn4 -- b/RConn1
  Current and Voltage Sensor (Three-Phase)/RConn3 -- a/RConn1
  Current and Voltage Sensor (Three-Phase)/LConn3 -- C/RConn1
  Current and Voltage Sensor (Three-Phase)/LConn1 -- A/RConn1
  Current and Voltage Sensor (Three-Phase)/LConn2 -- B/RConn1

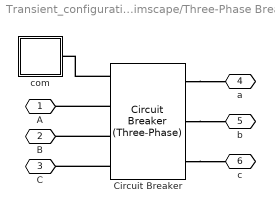
== system Transient_configuration_example_50_simscape/Three-Phase Breaker ==
  Circuit Breaker : ee_lib/Switches & Breakers/Circuit Breaker (Three-Phase)  port_option=ee.enum.threePhasePort.expanded  control_port_option=ee.enum.controlport.ps  R_closed=1e-08 Ohm  G_open=Three_PhaseBreaker_class('open',1000000,Inf,0.166666666666667,'off').objParamMappingDerived.NewDerivedParam.G_open 1/Ohm  threshold=0.5 V  breaker_behavior=ee.enum.switches.breakerBehavior.zeroCrossingEnable  i_th=1e-8 A
  com : Subsystem
  A : PMIOPort  Side=Left
  B : PMIOPort  Port=2  Side=Left
  C : PMIOPort  Port=3  Side=Left
  a : PMIOPort  Port=4  Side=Right
  b : PMIOPort  Port=5  Side=Right
  c : PMIOPort  Port=6  Side=Right
  connections:
  Circuit Breaker/LConn1 -- com/RConn1
  Circuit Breaker/LConn2 -- A/RConn1
  Circuit Breaker/LConn3 -- B/RConn1
  Circuit Breaker/LConn4 -- C/RConn1
  Circuit Breaker/RConn1 -- a/RConn1
  Circuit Breaker/RConn2 -- b/RConn1
  Circuit Breaker/RConn3 -- c/RConn1

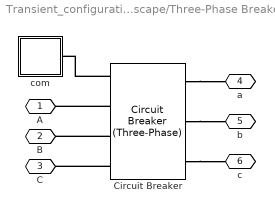
== system Transient_configuration_example_50_simscape/Three-Phase Breaker1 ==
  Circuit Breaker : ee_lib/Switches & Breakers/Circuit Breaker (Three-Phase)  port_option=ee.enum.threePhasePort.expanded  control_port_option=ee.enum.controlport.ps  R_closed=1e-08 Ohm  G_open=Three_PhaseBreaker_class('closed',1000000,Inf,0.99,'off').objParamMappingDerived.NewDerivedParam.G_open 1/Ohm  threshold=0.5 V  breaker_behavior=ee.enum.switches.breakerBehavior.zeroCrossingEnable  i_th=1e-8 A
  com : Subsystem
  A : PMIOPort  Side=Left
  B : PMIOPort  Port=2  Side=Left
  C : PMIOPort  Port=3  Side=Left
  a : PMIOPort  Port=4  Side=Right
  b : PMIOPort  Port=5  Side=Right
  c : PMIOPort  Port=6  Side=Right
  connections:
  Circuit Breaker/LConn1 -- com/RConn1
  Circuit Breaker/LConn2 -- A/RConn1
  Circuit Breaker/LConn3 -- B/RConn1
  Circuit Breaker/LConn4 -- C/RConn1
  Circuit Breaker/RConn1 -- a/RConn1
  Circuit Breaker/RConn2 -- b/RConn1
  Circuit Breaker/RConn3 -- c/RConn1

== system Transient_configuration_example_50_simscape/Three-Phase Fault ==
  Circuit Breaker (Three-Phase) : ee_lib/Switches & Breakers/Circuit Breaker (Three-Phase)  port_option=ee.enum.threePhasePort.expanded  control_port_option=ee.enum.controlport.ps  R_closed=1e-14 Ohm  G_open=Three_PhaseFault_class(1,0,NaN,1e-13,1e-07,Inf,'on','off').objParamMappingDerived.NewDerivedParam.G_open 1/Ohm  threshold=0.5 V  breaker_behavior=ee.enum.switches.breakerBehavior.zeroCrossingEnable  i_th=1e-8 A
  Electrical Reference : fl_lib/Electrical/Electrical Elements/Electrical Reference
  Rg : fl_lib/Electrical/Electrical Elements/Resistor  R=Three_PhaseFault_class(1,0,NaN,1e-13,1e-07,Inf,'on','off').objParamMappingDerived.NewDerivedParam.R_ng_fault Ohm  i_specify=off  i_priority=None  i=0 A  i_nominal_specify=off  i_nominal_value=1  i_nominal_unit=A  v_specify=off  v_priority=None  v=0 V  v_nominal_specify=off  v_nominal_value=1  v_nominal_unit=V
  com : Subsystem
  A : PMIOPort  Side=Left
  B : PMIOPort  Port=2  Side=Left
  C : PMIOPort  Port=3  Side=Left
  connections:
  com/RConn1 -- Circuit Breaker (Three-Phase)/LConn1
  Electrical Reference/LConn1 -- Rg/RConn1
  Rg/LConn1 -- Circuit Breaker (Three-Phase)/RConn1 -- Circuit Breaker (Three-Phase)/RConn2 -- Circuit Breaker (Three-Phase)/RConn3
  A/RConn1 -- Circuit Breaker (Three-Phase)/LConn2
  B/RConn1 -- Circuit Breaker (Three-Phase)/LConn3
  C/RConn1 -- Circuit Breaker (Three-Phase)/LConn4

== system Transient_configuration_example_50_simscape/Three-Phase Transformer Inductance Matrix Type (Two Windings) ==
  Two-Winding Transformer (Three-Phase) : ee_lib/Passive/Transformers/Two-Winding Transformer (Three-Phase)  SRated=150000000 V*A  FRated=60 Hz  Winding1Connection=3  VRated1=150000 V  Winding2Connection=3  VRated2=10000 V  CoreType=2  pu_Rw1=Three_PhaseTransformer_1_class('Yg','Yg',[150000000 60],[150000 10000],[1e-10 1e-11],10,1,0.04,100,1500,0.03).objParamMappingDerived.NewDerivedParam.pu_Rw1  pu_Rw2=Three_PhaseTransformer_1_class('Yg','Yg',[150000000 60],[150000 10000],[1e-10 1e-11],10,1,0.04,100,1500,0.03).objParamMappingDerived.NewDerivedParam.pu_Rw2  leakage_reactance_option=ee.enum.transformer_leakage.include  pu_Xl1=Three_PhaseTransformer_1_class('Yg','Yg',[150000000 60],[150000 10000],[1e-10 1e-11],10,1,0.04,100,1500,0.03).objParamMappingDerived.NewDerivedParam.pu_Xl1  pu_Xl2=Three_PhaseTransformer_1_class('Yg','Yg',[150000000 60],[150000 10000],[1e-10 1e-11],10,1,0.04,100,1500,0.03).objParamMappingDerived.NewDerivedParam.pu_Xl2  magnetizing_resistance_option=ee.enum.transformer_magnetizingResistance.include  pu_Rm=Three_PhaseTransformer_1_class('Yg','Yg',[150000000 60],[150000 10000],[1e-10 1e-11],10,1,0.04,100,1500,0.03).objParamMappingDerived.NewDerivedParam.pu_Rm  magnetizing_reactance_option=ee.enum.transformer_magnetizingReactance.include  saturation_option=ee.enum.transformer_saturation.exclude  pu_Xm=Three_PhaseTransformer_1_class('Yg','Yg',[150000000 60],[150000 10000],[1e-10 1e-11],10,1,0.04,100,1500,0.03).objParamMappingDerived.NewDerivedParam.pu_Xm  current_data=[0, .002, 1, 2]  magnetic_flux_data=[0, 1.2, 1.5, 1.51]  pu_X0=Three_PhaseTransformer_1_class('Yg','Yg',[150000000 60],[150000 10000],[1e-10 1e-11],10,1,0.04,100,1500,0.03).objParamMappingDerived.NewDerivedParam.pu_X0  i1_specify=off  i1_priority=None  i1=[ 0 0 0 ] A  i1_nominal_specify=off  i1_nominal_value=1  i1_nominal_unit=A  i2_specify=off  i2_priority=None  i2=[ 0 0 0 ] A  i2_nominal_specify=off  i2_nominal_value=1  i2_nominal_unit=A  phi_specify=off  phi_priority=None  phi=[ 0 0 0 ]  phi_nominal_specify=off  phi_nominal_value=1  phi_nominal_unit=1
  A : PMIOPort  Side=Left
  B : PMIOPort  Port=2  Side=Left
  C : PMIOPort  Port=3  Side=Left
  a : PMIOPort  Port=4  Side=Right
  b : PMIOPort  Port=5  Side=Right
  c : PMIOPort  Port=6  Side=Right
  connections:
  Two-Winding Transformer (Three-Phase)/RConn2 -- b/RConn1
  Two-Winding Transformer (Three-Phase)/RConn1 -- a/RConn1
  Two-Winding Transformer (Three-Phase)/RConn3 -- c/RConn1
  C/RConn1 -- Two-Winding Transformer (Three-Phase)/LConn3
  B/RConn1 -- Two-Winding Transformer (Three-Phase)/LConn2
  A/RConn1 -- Two-Winding Transformer (Three-Phase)/LConn1

== system Transient_configuration_example_50_simscape/Three-Phase Transformer Inductance Matrix Type (Two Windings)1 ==
  Two-Winding Transformer (Three-Phase) : ee_lib/Passive/Transformers/Two-Winding Transformer (Three-Phase)  SRated=150000000 V*A  FRated=60 Hz  Winding1Connection=3  VRated1=150000 V  Winding2Connection=3  VRated2=10000 V  CoreType=2  pu_Rw1=Three_PhaseTransformer_1_class('Yg','Yg',[150000000 60],[150000 10000],[1e-10 1e-11],10,1,0.04,100,1500,0.03).objParamMappingDerived.NewDerivedParam.pu_Rw1  pu_Rw2=Three_PhaseTransformer_1_class('Yg','Yg',[150000000 60],[150000 10000],[1e-10 1e-11],10,1,0.04,100,1500,0.03).objParamMappingDerived.NewDerivedParam.pu_Rw2  leakage_reactance_option=ee.enum.transformer_leakage.include  pu_Xl1=Three_PhaseTransformer_1_class('Yg','Yg',[150000000 60],[150000 10000],[1e-10 1e-11],10,1,0.04,100,1500,0.03).objParamMappingDerived.NewDerivedParam.pu_Xl1  pu_Xl2=Three_PhaseTransformer_1_class('Yg','Yg',[150000000 60],[150000 10000],[1e-10 1e-11],10,1,0.04,100,1500,0.03).objParamMappingDerived.NewDerivedParam.pu_Xl2  magnetizing_resistance_option=ee.enum.transformer_magnetizingResistance.include  pu_Rm=Three_PhaseTransformer_1_class('Yg','Yg',[150000000 60],[150000 10000],[1e-10 1e-11],10,1,0.04,100,1500,0.03).objParamMappingDerived.NewDerivedParam.pu_Rm  magnetizing_reactance_option=ee.enum.transformer_magnetizingReactance.include  saturation_option=ee.enum.transformer_saturation.exclude  pu_Xm=Three_PhaseTransformer_1_class('Yg','Yg',[150000000 60],[150000 10000],[1e-10 1e-11],10,1,0.04,100,1500,0.03).objParamMappingDerived.NewDerivedParam.pu_Xm  current_data=[0, .002, 1, 2]  magnetic_flux_data=[0, 1.2, 1.5, 1.51]  pu_X0=Three_PhaseTransformer_1_class('Yg','Yg',[150000000 60],[150000 10000],[1e-10 1e-11],10,1,0.04,100,1500,0.03).objParamMappingDerived.NewDerivedParam.pu_X0  i1_specify=off  i1_priority=None  i1=[ 0 0 0 ] A  i1_nominal_specify=off  i1_nominal_value=1  i1_nominal_unit=A  i2_specify=off  i2_priority=None  i2=[ 0 0 0 ] A  i2_nominal_specify=off  i2_nominal_value=1  i2_nominal_unit=A  phi_specify=off  phi_priority=None  phi=[ 0 0 0 ]  phi_nominal_specify=off  phi_nominal_value=1  phi_nominal_unit=1
  A : PMIOPort  Side=Left
  B : PMIOPort  Port=2  Side=Left
  C : PMIOPort  Port=3  Side=Left
  a : PMIOPort  Port=4  Side=Right
  b : PMIOPort  Port=5  Side=Right
  c : PMIOPort  Port=6  Side=Right
  connections:
  Two-Winding Transformer (Three-Phase)/RConn2 -- b/RConn1
  Two-Winding Transformer (Three-Phase)/RConn1 -- a/RConn1
  Two-Winding Transformer (Three-Phase)/RConn3 -- c/RConn1
  C/RConn1 -- Two-Winding Transformer (Three-Phase)/LConn3
  B/RConn1 -- Two-Winding Transformer (Three-Phase)/LConn2
  A/RConn1 -- Two-Winding Transformer (Three-Phase)/LConn1

== system Transient_configuration_example_50_simscape/|V2| ==
  Electrical Reference : fl_lib/Electrical/Electrical Elements/Electrical Reference
  Voltage Source : ee_lib/Sources/Voltage Source (Three-Phase)  vline_rms=10072 V  shift=14.2825 deg  freq=60 Hz  impedance_option=3  SShortCircuit=100000000 V*A  XR=7  R=Three_PhaseSource_class(10072,60,0,0.00026525198938992,100000000,10000,7,'on','off').objParamMappingDerived.NewDerivedParam.R Ohm  L=Three_PhaseSource_class(10072,60,0,0.00026525198938992,100000000,10000,7,'on','off').objParamMappingDerived.NewDerivedParam.L H  harmonic_option=0  harmonic_orders=[5, 7, 11, 13]  harmonic_ratios=[.1, .1, .1, .1]  G_parasitic=0 1/Ohm  I_specify=off  I_priority=None  I=[ 0 0 0 ] A  I_nominal_specify=off  I_nominal_value=1  I_nominal_unit=A
  A : PMIOPort  Side=Right
  B : PMIOPort  Port=2  Side=Right
  C : PMIOPort  Port=3  Side=Right
  connections:
  Voltage Source/RConn2 -- B/RConn1
  Voltage Source/RConn1 -- A/RConn1
  Voltage Source/RConn3 -- C/RConn1
  Electrical Reference/LConn1 -- Voltage Source/LConn1

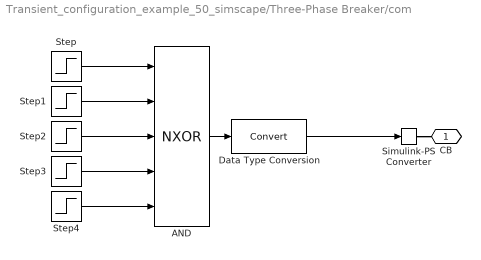
== system Transient_configuration_example_50_simscape/Three-Phase Breaker/com ==
  AND : Logic  Operator=NXOR  Inputs=5  IconShape=distinctive  AllPortsSameDT=off  OutDataTypeStr=boolean
  Data Type Conversion : DataTypeConversion  SaturateOnIntegerOverflow=off  RndMeth=Floor
  Simulink-PS Converter : nesl_utility/Simulink-PS Converter  PhysicalDomain=network_engine_domain  SubClassName=ps_input  LeftPortType=input  RightPortType=output  PseudoPeriodic=off  Frequencies=[]  NoiseDistribution=none  NoiseParameters=[]  Unit=1  AffineConversion=off  FilteringAndDerivatives=provide  SimscapeFilterOrder=1  InputFilterTimeConstant=0.001  UdotUserProvided=0
  Step : Step  Time=Three_PhaseBreaker_class('open',1000000,Inf,0.166666666666667,'off').objParamMappingDerived.NewDerivedParam.switchTime1  SampleTime=0
  Step1 : Step  Time=Three_PhaseBreaker_class('open',1000000,Inf,0.166666666666667,'off').objParamMappingDerived.NewDerivedParam.switchTime2  SampleTime=0
  Step2 : Step  Time=Three_PhaseBreaker_class('open',1000000,Inf,0.166666666666667,'off').objParamMappingDerived.NewDerivedParam.switchTime3  SampleTime=0
  Step3 : Step  Time=Three_PhaseBreaker_class('open',1000000,Inf,0.166666666666667,'off').objParamMappingDerived.NewDerivedParam.switchTime4  SampleTime=0
  Step4 : Step  Time=Three_PhaseBreaker_class('open',1000000,Inf,0.166666666666667,'off').objParamMappingDerived.NewDerivedParam.switchTime5  SampleTime=0
  CB : PMIOPort  Side=Right
  wires:
  Data Type Conversion/1 -> Simulink-PS Converter/1
  Step4/1 -> AND/5
  AND/1 -> Data Type Conversion/1
  Step3/1 -> AND/4
  Step1/1 -> AND/2
  Step/1 -> AND/1
  Step2/1 -> AND/3
  connections:
  Simulink-PS Converter/RConn1 -- CB/RConn1

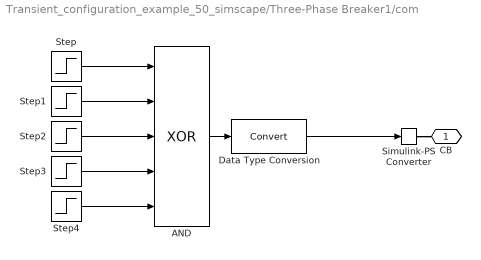
== system Transient_configuration_example_50_simscape/Three-Phase Breaker1/com ==
  AND : Logic  Operator=XOR  Inputs=5  IconShape=distinctive  AllPortsSameDT=off  OutDataTypeStr=boolean
  Data Type Conversion : DataTypeConversion  SaturateOnIntegerOverflow=off  RndMeth=Floor
  Simulink-PS Converter : nesl_utility/Simulink-PS Converter  PhysicalDomain=network_engine_domain  SubClassName=ps_input  LeftPortType=input  RightPortType=output  PseudoPeriodic=off  Frequencies=[]  NoiseDistribution=none  NoiseParameters=[]  Unit=1  AffineConversion=off  FilteringAndDerivatives=provide  SimscapeFilterOrder=1  InputFilterTimeConstant=0.001  UdotUserProvided=0
  Step : Step  Time=Three_PhaseBreaker_class('closed',1000000,Inf,0.99,'off').objParamMappingDerived.NewDerivedParam.switchTime1  SampleTime=0
  Step1 : Step  Time=Three_PhaseBreaker_class('closed',1000000,Inf,0.99,'off').objParamMappingDerived.NewDerivedParam.switchTime2  SampleTime=0
  Step2 : Step  Time=Three_PhaseBreaker_class('closed',1000000,Inf,0.99,'off').objParamMappingDerived.NewDerivedParam.switchTime3  SampleTime=0
  Step3 : Step  Time=Three_PhaseBreaker_class('closed',1000000,Inf,0.99,'off').objParamMappingDerived.NewDerivedParam.switchTime4  SampleTime=0
  Step4 : Step  Time=Three_PhaseBreaker_class('closed',1000000,Inf,0.99,'off').objParamMappingDerived.NewDerivedParam.switchTime5  SampleTime=0
  CB : PMIOPort  Side=Right
  wires:
  Data Type Conversion/1 -> Simulink-PS Converter/1
  Step4/1 -> AND/5
  AND/1 -> Data Type Conversion/1
  Step3/1 -> AND/4
  Step1/1 -> AND/2
  Step/1 -> AND/1
  Step2/1 -> AND/3
  connections:
  Simulink-PS Converter/RConn1 -- CB/RConn1

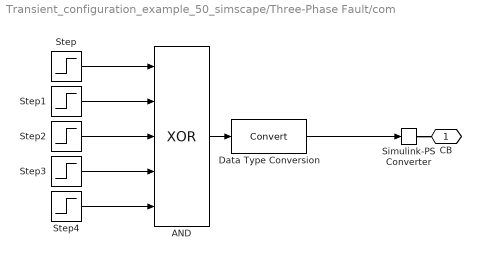
== system Transient_configuration_example_50_simscape/Three-Phase Fault/com ==
  AND : Logic  Operator=XOR  Inputs=5  IconShape=distinctive  AllPortsSameDT=off  OutDataTypeStr=boolean
  Data Type Conversion : DataTypeConversion  SaturateOnIntegerOverflow=off  RndMeth=Floor
  Simulink-PS Converter : nesl_utility/Simulink-PS Converter  PhysicalDomain=network_engine_domain  SubClassName=ps_input  LeftPortType=input  RightPortType=output  PseudoPeriodic=off  Frequencies=[]  NoiseDistribution=none  NoiseParameters=[]  Unit=1  AffineConversion=off  FilteringAndDerivatives=provide  SimscapeFilterOrder=1  InputFilterTimeConstant=0.001  UdotUserProvided=0
  Step : Step  Time=Three_PhaseFault_class(1,0,NaN,1e-13,1e-07,Inf,'on','off').objParamMappingDerived.NewDerivedParam.switchTime1  SampleTime=0
  Step1 : Step  Time=Three_PhaseFault_class(1,0,NaN,1e-13,1e-07,Inf,'on','off').objParamMappingDerived.NewDerivedParam.switchTime2  SampleTime=0
  Step2 : Step  Time=Three_PhaseFault_class(1,0,NaN,1e-13,1e-07,Inf,'on','off').objParamMappingDerived.NewDerivedParam.switchTime3  SampleTime=0
  Step3 : Step  Time=Three_PhaseFault_class(1,0,NaN,1e-13,1e-07,Inf,'on','off').objParamMappingDerived.NewDerivedParam.switchTime4  SampleTime=0
  Step4 : Step  Time=Three_PhaseFault_class(1,0,NaN,1e-13,1e-07,Inf,'on','off').objParamMappingDerived.NewDerivedParam.switchTime5  SampleTime=0
  CB : PMIOPort  Side=Right
  wires:
  Step2/1 -> AND/3
  Step/1 -> AND/1
  Step1/1 -> AND/2
  Step3/1 -> AND/4
  AND/1 -> Data Type Conversion/1
  Step4/1 -> AND/5
  Data Type Conversion/1 -> Simulink-PS Converter/1
  connections:
  Simulink-PS Converter/RConn1 -- CB/RConn1
